simulink model "PID"  (R2018a)
settings: Solver=VariableStepAuto  StartTime=0.0  StopTime=10.0  RelTol=1e-3
settings Model: Creator=misar  LastModifiedBy=misar

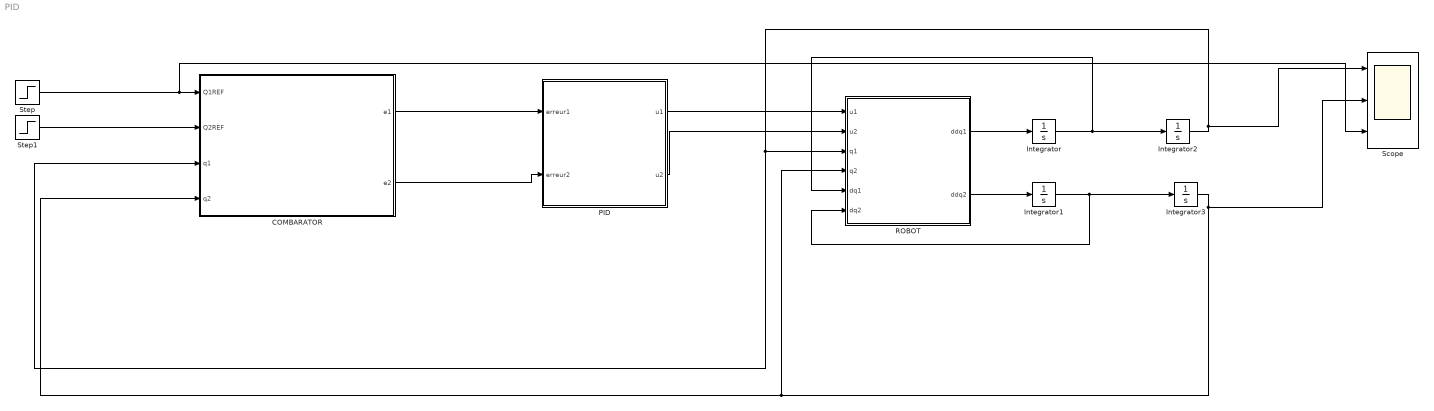
== system PID ==
  "COMBARATOR " : Subsystem
  Integrator{,1..3} (4 alike) : Integrator
  "PID " : Subsystem
  "ROBOT " : Subsystem
  Scope : Scope  NumInputPorts=3
  Step : Step  SampleTime=0
  Step1 : Step  SampleTime=0
  wires:
  "ROBOT "/1(ddq1) -> Integrator/1
  "ROBOT "/2(ddq2) -> Integrator1/1
  Integrator/1 -> "ROBOT "/5(dq1), Integrator2/1
  Integrator1/1 -> "ROBOT "/6(dq2), Integrator3/1
  "PID "/1(u1) -> "ROBOT "/1(u1)
  "PID "/2(u2) -> "ROBOT "/2(u2)
  Step1/1 -> "COMBARATOR "/2(Q2REF)
  "COMBARATOR "/1(e1) -> "PID "/1(erreur1)
  "COMBARATOR "/2(e2) -> "PID "/2(erreur2)
  Integrator2/1 -> Scope/1, "COMBARATOR "/3("q1 "), "ROBOT "/3(q1)
  Integrator3/1 -> Scope/2, "COMBARATOR "/4("q2 "), "ROBOT "/4(q2)
  Step/1 -> Scope/3, "COMBARATOR "/1(Q1REF)

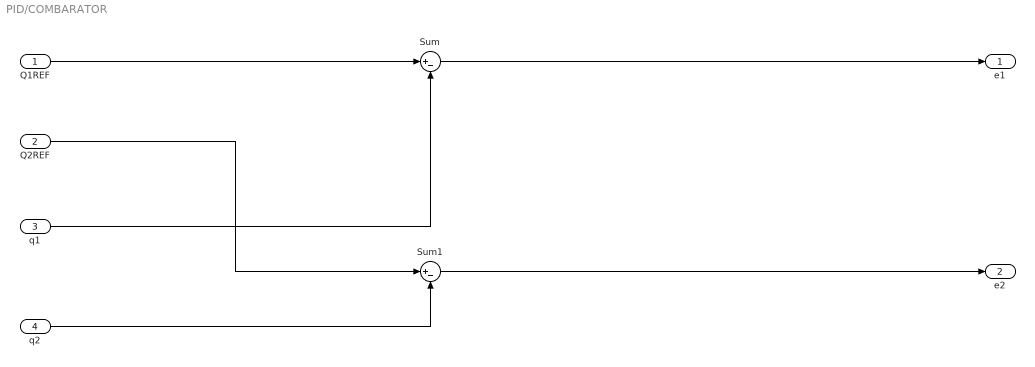
== system PID/COMBARATOR  ==
  Q1REF : Inport
  Q2REF : Inport  Port=2
  "q1 " : Inport  Port=3
  "q2 " : Inport  Port=4
  Sum : Sum  Inputs=|+-
  Sum1 : Sum  Inputs=|+-
  e1 : Outport
  e2 : Outport  Port=2
  wires:
  Q1REF/1 -> Sum/1
  "q1 "/1 -> Sum/2
  Q2REF/1 -> Sum1/1
  "q2 "/1 -> Sum1/2
  Sum/1 -> e1/1
  Sum1/1 -> e2/1

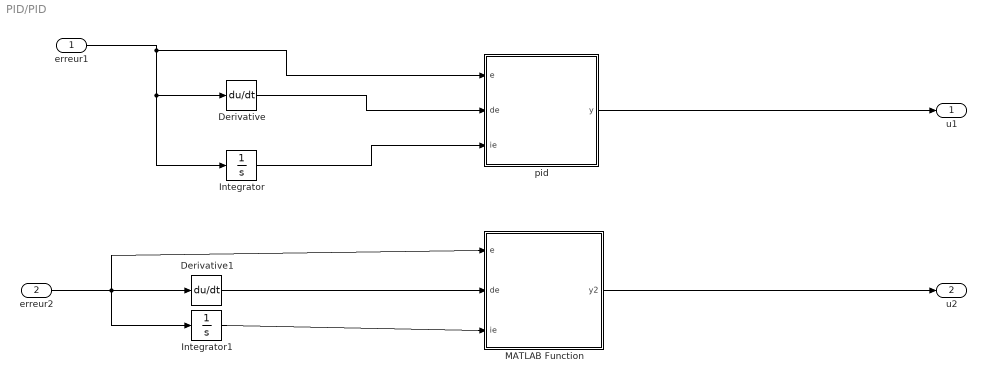
== system PID/PID  ==
  erreur1 : Inport
  erreur2 : Inport  Port=2
  Derivative : Derivative
  Derivative1 : Derivative
  Integrator : Integrator
  Integrator1 : Integrator
  MATLAB Function : MATLAB Function  TreatAsAtomicUnit=on
  "pid " : MATLAB Function  TreatAsAtomicUnit=on
  u1 : Outport
  u2 : Outport  Port=2
  wires:
  erreur1/1 -> "pid "/1(e), Integrator/1, Derivative/1
  Derivative/1 -> "pid "/2(de)
  Integrator/1 -> "pid "/3(ie)
  Derivative1/1 -> MATLAB Function/2(de)
  Integrator1/1 -> MATLAB Function/3(ie)
  erreur2/1 -> MATLAB Function/1(e), Integrator1/1, Derivative1/1
  "pid "/1(y) -> u1/1
  MATLAB Function/1(y2) -> u2/1

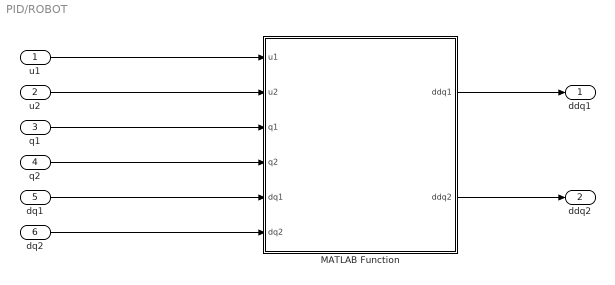
== system PID/ROBOT  ==
  u1 : Inport
  u2 : Inport  Port=2
  q1 : Inport  Port=3
  q2 : Inport  Port=4
  dq1 : Inport  Port=5
  dq2 : Inport  Port=6
  MATLAB Function : MATLAB Function  TreatAsAtomicUnit=on
  ddq1 : Outport
  ddq2 : Outport  Port=2
  wires:
  u1/1 -> MATLAB Function/1(u1)
  u2/1 -> MATLAB Function/2(u2)
  q1/1 -> MATLAB Function/3(q1)
  q2/1 -> MATLAB Function/4(q2)
  dq2/1 -> MATLAB Function/6(dq2)
  dq1/1 -> MATLAB Function/5(dq1)
  MATLAB Function/1(ddq1) -> ddq1/1
  MATLAB Function/2(ddq2) -> ddq2/1

== matlab function PID/PID /pid  ==
  data: e input; y output; de input; ie input
function y = PID(e,de,ie)
kp=100;
ki=2;
kd=3;

y = kp*e+kd*de+ki*ie;
end

== matlab function PID/PID /MATLAB Function ==
  data: e input; y2 output; de input; ie input
function y2 = PID(e,de,ie)
kp=100;
ki=2;
kd=3;

y2 = kp*e+kd*de+ki*ie;
end

== matlab function PID/ROBOT /MATLAB Function ==
  data: u1 input; ddq1 output; u2 input; q1 input; q2 input; dq1 input; dq2 input; ddq2 output
function [ddq1,ddq2] = fcn(u1,u2,q1,q2,dq1,dq2)
m1=0.5;
m2=0.5;
a1=0.5;
a2=0.5;
A=0.5;
g=10;
ddq=[ddq1 ddq2]'; 
dq=[dq1 dq2]';
u=[u1 u2]';
D=[m1 m2-(m2/2)*q2*cos(q2) ; -0.5*m2*q2*cos(q1) A+(m2*a2*a2)/4];
c=[0 0.5*m2*q2*sin(q2)*dq2;0 0];
v=[g(m1+m2)  g*(-m2*a2/2*cos(q2))];
ddq2=inv(D)*(u-c*dq-v);
ddq1=inv(D)*(u-c*dq-v);
%ddq1(1),ddq2(2) ;
end
